simulink model "untitled"  (R2020a)
settings: Solver=VariableStepAuto  StartTime=0.0  StopTime=24  FixedStep=1e-6  MaxStep=1e-5  MinStep=1e-6  RelTol=1e-3
undefined symbols (not defined in the file): a, Acid, e_g, I_sc, k, Lead, N_p, N_s, q, R_s, R_sh, T_r, V_oc
libraries: powerlib x48, simulink x10, powerlib_meascontrol x6, electricdrivelib x1
settings Model: SimulationMode=accelerator  Creator=Tareeq  LastModifiedBy=Tareeq
settings SolverCC: AlgebraicLoopSolver=LineSearch

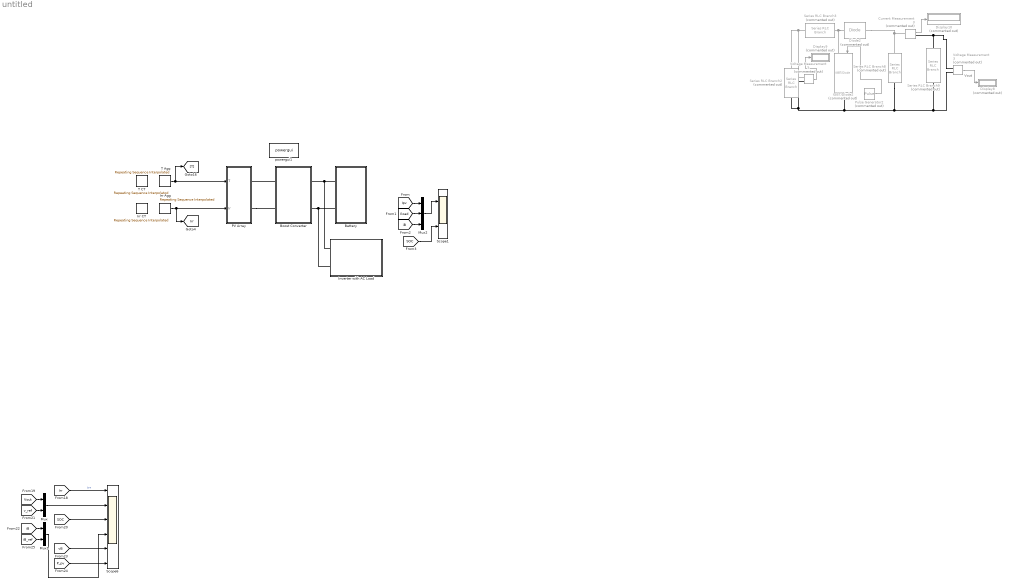
== system untitled ==
  note: Vout
  Battery : Subsystem
  Boost Converter : Subsystem
  Current Measurement3 : powerlib/Measurements/Current Measurement  Commented=on  PhasorSimulation=off  OutputType=Complex  PSBequivalent=0
  Diode2 : powerlib/Power Electronics/Diode  Commented=on  Ron=0.001  Lon=0  Vf=0.8  IC=0  UseSnubber=0  Rs=500  Cs=250e-9  Measurements=off
  Display10 : Display  Commented=on
  Display8 : Display  Commented=on
  Display9 : Display  Commented=on
  IGBT/Diode2 : powerlib/Power Electronics/IGBT//Diode  Commented=on  Ron=1e-3  Rs=inf  Cs=inf  Measurements=off
  Inverter with AC Load : Subsystem
  Irr Agg : simulink/Sources/Repeating Sequence Interpolated  OutValues="[0.412 0.412 0.395 0.395 0.407 0.407 0.332 0.332 0.375 0.375 0.384 0.384 0.345 0.345 0.994 0.994 462.1 462.1  804 804 922 922 973 973 996 996 1003 1003 1006 1006 988 988 881 881 828 828 338.9 338.9 240.5 240.5 0.015 0.015 0.119 0.119 0.375 0.375 0.291 0.291 ].'"  TimeValues=[0 1 1.01 2 2.01 3 3.01 4 4.01 5 5.01 6 6.01 7 7.01 8 8.01 9 9.01 10 10.01 11 11.01 12 12.01 13 13.01 14 14.01 15 15.01 16 16.01 17 17.01 18 18.01 19 19.01 20 20.01 21 21.01 22 22.02 23 23.01 24].'  LookUpMeth=Interpolation-Use End Values  tsamp=1e-5  OutMin=[]  OutMax=[]  OutDataTypeStr=double  OutputDataTypeScalingMode=double  OutDataType=fixdt(0,8)  OutScaling=2^-10
  Irr CT : simulink/Sources/Repeating Sequence Interpolated  OutValues=[0 0 0 0 0 0 0 0 0 0 2.6 2.6 53.2 53.2 151.6 151.6 270.1 270.1 383.6 383.6 450.5 450.5 480.4 480.4 474.3 474.3 443.6 443.6 375.2 375.2 288.4 288.4 200.3 200.3 122.3 122.3 61.3 61.3 14.1 14.1 0.1 0.1 0 0 0 0 0 0].'  TimeValues=[0 1 1.01 2 2.01 3 3.01 4 4.01 5 5.01 6 6.01 7 7.01 8 8.01 9 9.01 10 10.01 11 11.01 12 12.01 13 13.01 14 14.01 15 15.01 16 16.01 17 17.01 18 18.01 19 19.01 20 20.01 21 21.01 22 22.02 23 23.01 24].'  LookUpMeth=Interpolation-Use End Values  tsamp=1e-5  OutMin=[]  OutMax=[]  OutDataTypeStr=double  OutputDataTypeScalingMode=double  OutDataType=fixdt(0,8)  OutScaling=2^-10
  Mux : Mux  Inputs=2
  Mux1 : Mux  Inputs=2
  Mux2 : Mux  Inputs=3
  PV Array : Subsystem
  Pulse Generator2 : DiscretePulseGenerator  Commented=on  PulseType=Time based  Period=1/10000  PulseWidth=89
  Scope1 : Scope  NumInputPorts=2
  Scope6 : Scope  NumInputPorts=6
  Series RLC Branch2 : powerlib/Elements/Series RLC Branch  Commented=on  LConnTagsString=__new0  RConnTagsString=__new0  BranchType=C  Resistance=0.0001  Inductance=1e-3  SetiL0=off  InitialCurrent=0  Capacitance=2957.5e-6  Setx0=off  InitialVoltage=0  Measurements=None
  Series RLC Branch3 : powerlib/Elements/Series RLC Branch  Commented=on  LConnTagsString=__new0  RConnTagsString=__new0  BranchType=L  Resistance=0.0001  Inductance=153e-5  SetiL0=off  InitialCurrent=0  Capacitance=77.04e-6  Setx0=off  InitialVoltage=0  Measurements=None
  Series RLC Branch8 : powerlib/Elements/Series RLC Branch  Commented=on  LConnTagsString=__new0  RConnTagsString=__new0  BranchType=C  Resistance=0.0001  Inductance=780.60e-6  SetiL0=off  InitialCurrent=0  Capacitance=520.35e-6  Setx0=off  InitialVoltage=0  Measurements=None
  Series RLC Branch9 : powerlib/Elements/Series RLC Branch  Commented=on  LConnTagsString=__new0  RConnTagsString=__new0  BranchType=R  Resistance=173  Inductance=780.60e-6  SetiL0=off  InitialCurrent=0  Capacitance=2.09e-6  Setx0=off  InitialVoltage=0  Measurements=None
  T Agg : simulink/Sources/Repeating Sequence Interpolated  OutValues=[27.9 27.9 26.65 26.65 26.01 26.01 25.06 25.06 22.9 22.9 21.38 21.38 20.93 20.93 20.06 20.06 22.17 22.17 26.32 26.32 30.42 30.42 33.67 33.67 36.43 36.43 38.46 38.46 40.52 40.52 41.41 41.41 41.7 41.7 41.92 41.92 41.44 41.44 39.97 39.97 36.15 36.15 34.32 34.32 32.02 32.02 30.8 30.8].'  TimeValues=[0 1 1.01 2 2.01 3 3.01 4 4.01 5 5.01 6 6.01 7 7.01 8 8.01 9 9.01 10 10.01 11 11.01 12 12.01 13 13.01 14 14.01 15 15.01 16 16.01 17 17.01 18 18.01 19 19.01 20 20.01 21 21.01 22 22.01 23 23.01 24].'  LookUpMeth=Interpolation-Use End Values  tsamp=1e-5  OutMin=[]  OutMax=[]  OutDataTypeStr=double  OutputDataTypeScalingMode=double  OutDataType=fixdt(0,8)  OutScaling=2^-10
  T CT : simulink/Sources/Repeating Sequence Interpolated  OutValues=[16.07 16.07 15.8 15.8 15.52 15.52 15.29 15.29 15.07 15.07 14.88 14.88 14.88 14.88 15.39 15.39 16.53 16.53 18.11 18.11 19.4 19.4 20.28 20.28 20.79 20.79 21.08 21.08 21.21 21.21 21.10 21.10 20.72 20.72 19.98 19.98 18.88 18.88 17.94 17.94 17.35 17.35 16.99 16.99 16.65 16.65 16.35 16.35].'  TimeValues=[0 1 1.01 2 2.01 3 3.01 4 4.01 5 5.01 6 6.01 7 7.01 8 8.01 9 9.01 10 10.01 11 11.01 12 12.01 13 13.01 14 14.01 15 15.01 16 16.01 17 17.01 18 18.01 19 19.01 20 20.01 21 21.01 22 22.01 23 23.01 24].'  LookUpMeth=Interpolation-Use End Values  tsamp=1e-5  OutMin=[]  OutMax=[]  OutDataTypeStr=double  OutputDataTypeScalingMode=double  OutDataType=fixdt(0,8)  OutScaling=2^-10
  Voltage Measurement3 : powerlib/Measurements/Voltage Measurement  Commented=on  PhasorSimulation=off  OutputType=Complex  PSBequivalent=0
  Voltage Measurement5 : powerlib/Measurements/Voltage Measurement  Commented=on  PhasorSimulation=off  OutputType=Complex  PSBequivalent=0
  powergui1 : powerlib/powergui  Priority=1  SimulationMode=Continuous  SampleTime=1e-5  frequency=60  Iterations=50  frequencyindice=0  Pbase=100e6  ErrMax=1e-4  UnitsV=kV  UnitsW=MW  buscounter=0  FunctionMessages=off  echomessages=off  EnableUseOfTLC=off  CurrentSourceSwitches=off  DisableSnubberDevices=off  DisableRonSwitches=off  DisableVfSwitches=off  DisplayEquations=off  AutomaticDiscreteSolvers=off  SolverType=Tustin/Backward Euler (TBE)  Interpol=off  ExternalGateDelay=off  methode=off  Ts=100  x0status=blocks  SPID=on  SwTol=0  HookPort=off  NonlinearTolerance=1e-4  nMaxIteration=100  ContinueOnMaxIteration=off  RestoreLinks=warning  ResistiveCurrentMeasurement=off  Frange=[0:2:500]  Ylog=off  Xlog=on  ShowGrid=off  save=off  variable=ZData  structure=0  ZoomFFT=off  StartTime=0.0  cycles=1  DisplayStyle=1  fundamental=60  FreqAxis=off  MaxFrequency=1000  frequencyindicesteady=1  RmsSteady=1  display=off
  tag scope: Irr=global
  wires:
  [Irr] -> Scope6/1  "irr"
  [v_ref] -> Mux/2
  [iB] -> Mux1/1
  [iB_ref] -> Mux1/2
  [P_pv] -> Scope6/6
  Mux1/1 -> Scope6/4
  [SOC] -> Scope6/3
  Mux/1 -> Scope6/2
  [vB] -> Scope6/5
  [Vout] -> Mux/1
  Voltage Measurement5/1 -> Display9/1
  Voltage Measurement3/1 -> Display8/1
  Pulse Generator2/1 -> IGBT/Diode2/1
  Current Measurement3/1 -> Display10/1
  Irr Agg/1 -> [Irr], PV Array/2(Ir)
  T Agg/1 -> [T], PV Array/1(T)
  Mux2/1 -> Scope1/1
  [iB] -> Mux2/3
  [Iload] -> Mux2/2
  [Ipv] -> Mux2/1
  [SOC] -> Scope1/2
  connections:
  Current Measurement3/RConn1 -- Voltage Measurement3/LConn1 -- Series RLC Branch9/RConn1
  Series RLC Branch2/RConn1 -- Voltage Measurement5/LConn2 -- IGBT/Diode2/RConn1 -- Voltage Measurement3/LConn2 -- Series RLC Branch9/LConn1 -- Series RLC Branch8/RConn1
  Diode2/LConn1 -- Series RLC Branch3/LConn1 -- IGBT/Diode2/LConn1
  Diode2/RConn1 -- Series RLC Branch8/LConn1 -- Current Measurement3/LConn1
  Series RLC Branch3/RConn1 -- Voltage Measurement5/LConn1 -- Series RLC Branch2/LConn1
  Boost Converter/LConn1 -- PV Array/RConn1
  PV Array/RConn2 -- Boost Converter/LConn2
  Boost Converter/RConn2 -- Inverter with AC Load/LConn2 -- Battery/LConn2
  Boost Converter/RConn1 -- Inverter with AC Load/LConn1 -- Battery/LConn1

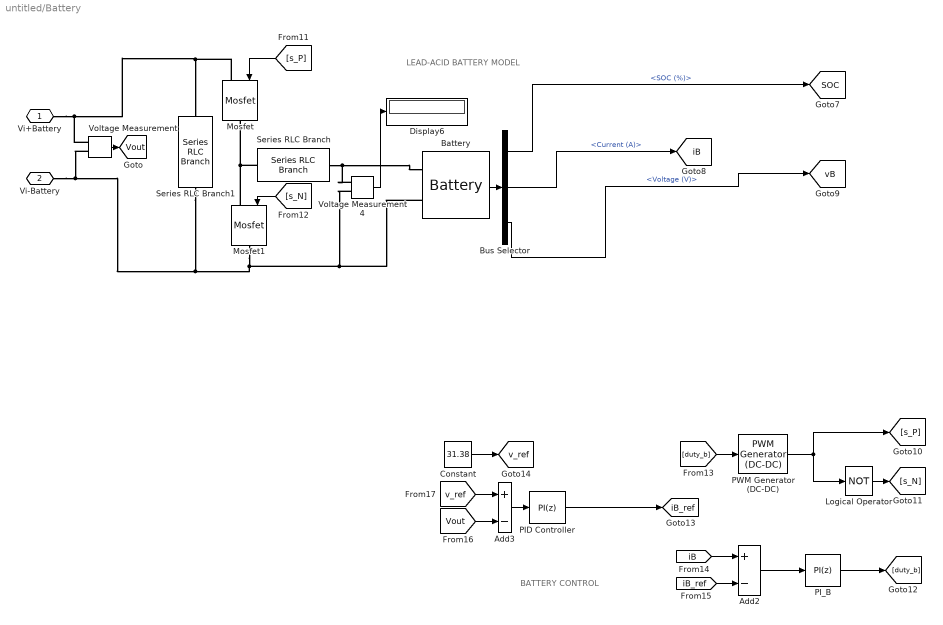
== system untitled/Battery ==
  note: LEAD-ACID BATTERY MODEL
  note: BATTERY CONTROL
  Add2 : Sum  Inputs=+-
  Add3 : Sum  Inputs=+-
  Battery : electricdrivelib/Extra Sources/Battery  BatType=Lead-Acid  ShowTempParam=off  ThermalPreset=no  ShowAgeParam=off  NomV=24  NomQ=400  SOC=100  Batt_Tr=1  PresetModel=on  MaxQ=416.6667  MinV=18  FullV=26.1316  Dis_rate=80  R=0.0006  Normal_OP=124.1111  expZone="[24.4342      1.33333]"  current=[6.5 13 32.5]  Units=Time  Tci=20  NomT=20  T2=-30  MaxQ2=4.8  FullV2=7.1  Normal_OP2=5.655  expZone2="[6.58           1]"  Rca=0.6  ti=2000  Dp=0  Neq0=0  Tsim=1e6  Ta1=25  Qeol=5.4*0.9  Reol=0.013333*1.2  Char_age=[2.3478, 3]  Dis_age=[2.3478, 10]  N1=1500  N2=10500  N3=1000  N4=1400  Ta2=45  N5=950
  Bus Selector : BusSelector  OutputSignals=SOC (%),Current (A),Voltage (V)
  Constant : Constant  Value=31.38
  Display6 : Display
  Logical Operator : Logic  Operator=NOT  Inputs=1  AllPortsSameDT=off  OutDataTypeStr=boolean
  Mosfet : powerlib/Power Electronics/Mosfet  Ron=0.1  Lon=0  Rd=0.01  Vfd=0  IC=0  Rs=1e5  Cs=inf  Measurements=off
  Mosfet1 : powerlib/Power Electronics/Mosfet  Ron=0.1  Lon=0  Rd=0.01  Vfd=0  IC=0  Rs=1e5  Cs=inf  Measurements=off
  PID Controller : simulink/Continuous/PID Controller  Controller=PI  Form=Parallel  TimeDomain=Discrete-time  UseExternalTs=off  SampleTime=50e-6  IntegratorMethod=Forward Euler  FilterMethod=Forward Euler  ControllerParametersSource=internal  P=0.05  I=100  D=0  UseFilter=on  N=100  TunerSelectOption=Transfer Function Based (PID Tuner App)  InitialConditionSource=internal  InitialConditionForIntegrator=1  InitialConditionForFilter=0  DifferentiatorICPrevScaledInput=0  ExternalReset=none  TrackingMode=off  Kt=1  LimitOutput=on  UpperSaturationLimit=80  LowerSaturationLimit=-80  LinearizeAsGain=on  AntiWindupMode=none  Kb=1  POutMin=[]  POutMax=[]  IOutMin=[]  IOutMax=[]  DOutMin=[]  DOutMax=[]  NOutMin=[]  NOutMax=[]  SumOutMin=[]  SumOutMax=[]  SaturationOutMin=[]  SaturationOutMax=[]  PParamMin=[]  PParamMax=[]  IParamMin=[]  IParamMax=[]  DParamMin=[]  DParamMax=[]  NParamMin=[]  NParamMax=[]  KbParamMin=[]  KbParamMax=[]  KtParamMin=[]  KtParamMax=[]  KbOutMin=[]  KbOutMax=[]  KtOutMin=[]  KtOutMax=[]  IntegratorOutMin=[]  IntegratorOutMax=[]  FilterOutMin=[]  FilterOutMax=[]  SumI1OutMin=[]  SumI1OutMax=[]  SumI2OutMin=[]  SumI2OutMax=[]  SumI3OutMin=[]  SumI3OutMax=[]  SumI4OutMin=[]  SumI4OutMax=[]  SumDOutMin=[]  SumDOutMax=[]  DifferentiatorOutMin=[]  DifferentiatorOutMax=[]  FilterDiffOutCoefMin=[]  FilterDiffOutCoefMax=[]  ReciprocalOutMin=[]  ReciprocalOutMax=[]  SumDenOutMin=[]  SumDenOutMax=[]  SumNumOutMin=[]  SumNumOutMax=[]  DivideOutMin=[]  DivideOutMax=[]  UdiffTsProdOutMin=[]  UdiffTsProdOutMax=[]  NTsProdOutMin=[]  NTsProdOutMax=[]  UintegralTsProdOutMin=[]  UintegralTsProdOutMax=[]  UngainTsProdOutMin=[]  UngainTsProdOutMax=[]  IntegratorContinuousStateAttributes=''  IntegratorStateMustResolveToSignalObject=off  IntegratorRTWStateStorageClass=Auto  FilterContinuousStateAttributes=''  FilterStateMustResolveToSignalObject=off  FilterRTWStateStorageClass=Auto  ParallelPVariant=InternalParameters  IdealPVariant=Disabled  IVariant=InternalParameters  DVariant=Disabled  IntegratorVariant=Discrete  SatVariant=Enabled  AWVariant=Passthrough  PCopyVariant=Disabled  TRVariant=Disabled  FdbkBlocksVariant=Forward  IdealPFdbkVariant=Disabled  SatFdbkVariant=Disabled  DerivativeFilterVariant=Disabled  NVariant=Disabled  NCopyVariant=Disabled_SignalSpec  FilterICVariant=Disabled  IntegratorICVariant=InternalICs  ExternalResetVariant=Disabled  TRSumVariant=Passthrough  SumFdbkVariant=Disabled  SumVariant=Sum_PI  TsampFilterVariant=InternalTs  TsampNgainVariant=Passthrough  TsampIntegralVariant=Passthrough
  PI_B : simulink/Continuous/PID Controller  Controller=PI  Form=Parallel  TimeDomain=Discrete-time  UseExternalTs=off  SampleTime=1e-5  IntegratorMethod=Forward Euler  FilterMethod=Forward Euler  ControllerParametersSource=internal  P=0.5  I=10  D=0  UseFilter=on  N=100  TunerSelectOption=Transfer Function Based (PID Tuner App)  InitialConditionSource=internal  InitialConditionForIntegrator=0  InitialConditionForFilter=0  DifferentiatorICPrevScaledInput=0  ExternalReset=none  TrackingMode=off  Kt=1  LimitOutput=on  UpperSaturationLimit=1  LowerSaturationLimit=0  LinearizeAsGain=off  AntiWindupMode=none  Kb=1  POutMin=[]  POutMax=[]  IOutMin=[]  IOutMax=[]  DOutMin=[]  DOutMax=[]  NOutMin=[]  NOutMax=[]  SumOutMin=[]  SumOutMax=[]  SaturationOutMin=[]  SaturationOutMax=[]  PParamMin=[]  PParamMax=[]  IParamMin=[]  IParamMax=[]  DParamMin=[]  DParamMax=[]  NParamMin=[]  NParamMax=[]  KbParamMin=[]  KbParamMax=[]  KtParamMin=[]  KtParamMax=[]  KbOutMin=[]  KbOutMax=[]  KtOutMin=[]  KtOutMax=[]  IntegratorOutMin=[]  IntegratorOutMax=[]  FilterOutMin=[]  FilterOutMax=[]  SumI1OutMin=[]  SumI1OutMax=[]  SumI2OutMin=[]  SumI2OutMax=[]  SumI3OutMin=[]  SumI3OutMax=[]  SumI4OutMin=[]  SumI4OutMax=[]  SumDOutMin=[]  SumDOutMax=[]  DifferentiatorOutMin=[]  DifferentiatorOutMax=[]  FilterDiffOutCoefMin=[]  FilterDiffOutCoefMax=[]  ReciprocalOutMin=[]  ReciprocalOutMax=[]  SumDenOutMin=[]  SumDenOutMax=[]  SumNumOutMin=[]  SumNumOutMax=[]  DivideOutMin=[]  DivideOutMax=[]  UdiffTsProdOutMin=[]  UdiffTsProdOutMax=[]  NTsProdOutMin=[]  NTsProdOutMax=[]  UintegralTsProdOutMin=[]  UintegralTsProdOutMax=[]  UngainTsProdOutMin=[]  UngainTsProdOutMax=[]  IntegratorContinuousStateAttributes=''  IntegratorStateMustResolveToSignalObject=off  IntegratorRTWStateStorageClass=Auto  FilterContinuousStateAttributes=''  FilterStateMustResolveToSignalObject=off  FilterRTWStateStorageClass=Auto  ParallelPVariant=InternalParameters  IdealPVariant=Disabled  IVariant=InternalParameters  DVariant=Disabled  IntegratorVariant=Discrete  SatVariant=Enabled  AWVariant=Passthrough  PCopyVariant=Disabled  TRVariant=Disabled  FdbkBlocksVariant=Forward  IdealPFdbkVariant=Disabled  SatFdbkVariant=Disabled  DerivativeFilterVariant=Disabled  NVariant=Disabled  NCopyVariant=Disabled_SignalSpec  FilterICVariant=Disabled  IntegratorICVariant=InternalICs  ExternalResetVariant=Disabled  TRSumVariant=Passthrough  SumFdbkVariant=Disabled  SumVariant=Sum_PI  TsampFilterVariant=InternalTs  TsampNgainVariant=Passthrough  TsampIntegralVariant=Passthrough
  PWM Generator (DC-DC) : powerlib_meascontrol/Pulse & Signal Generators/PWM Generator (DC-DC)  Fsw=10e3  Ts=1e-5
  Series RLC Branch : powerlib/Elements/Series RLC Branch  LConnTagsString=__new0  RConnTagsString=__new0  BranchType=RL  Resistance=0.005  Inductance=5.76e-4  SetiL0=off  InitialCurrent=0  Capacitance=0.5e-3  Setx0=off  InitialVoltage=0  Measurements=None
  Series RLC Branch1 : powerlib/Elements/Series RLC Branch  LConnTagsString=__new0  RConnTagsString=__new0  BranchType=RC  Resistance=1e-4  Inductance=780.60e-6  SetiL0=off  InitialCurrent=0  Capacitance=1e-6  Setx0=off  InitialVoltage=0  Measurements=None
  Voltage Measurement : powerlib/Measurements/Voltage Measurement  PhasorSimulation=off  OutputType=Complex  PSBequivalent=0
  Voltage Measurement4 : powerlib/Measurements/Voltage Measurement  PhasorSimulation=off  OutputType=Complex  PSBequivalent=0
  Vi+Battery : PMIOPort  Side=Left
  Vi-Battery : PMIOPort  Port=2  Side=Left
  tag scope: SOC=global, Vout=global, iB=global, iB_ref=global, vB=global, v_ref=global
  wires:
  Voltage Measurement4/1 -> Display6/1
  Bus Selector/3 -> [vB]  "<Voltage (V)>"
  [s_N] -> Mosfet1/1
  Bus Selector/2 -> [iB]  "<Current (A)>"
  [s_P] -> Mosfet/1
  Battery/1 -> Bus Selector/1
  [duty_b] -> PWM Generator (DC-DC)/1
  Constant/1 -> [v_ref]
  [iB] -> Add2/1
  [Vout] -> Add3/2
  [iB_ref] -> Add2/2
  Add3/1 -> PID Controller/1
  PI_B/1 -> [duty_b]
  [v_ref] -> Add3/1
  PWM Generator (DC-DC)/1 -> Logical Operator/1, [s_P]
  PID Controller/1 -> [iB_ref]
  Add2/1 -> PI_B/1
  Logical Operator/1 -> [s_N]
  Voltage Measurement/1 -> [Vout]
  Bus Selector/1 -> [SOC]  "<SOC (%)>"
  connections:
  Battery/LConn1 -- Series RLC Branch/RConn1 -- Voltage Measurement4/LConn1
  Mosfet/RConn1 -- Series RLC Branch/LConn1 -- Mosfet1/LConn1
  Mosfet/LConn1 -- Voltage Measurement/LConn1 -- Vi+Battery/RConn1 -- Series RLC Branch1/LConn1
  Battery/LConn2 -- Voltage Measurement/LConn2 -- Vi-Battery/RConn1 -- Series RLC Branch1/RConn1 -- Mosfet1/RConn1 -- Voltage Measurement4/LConn2

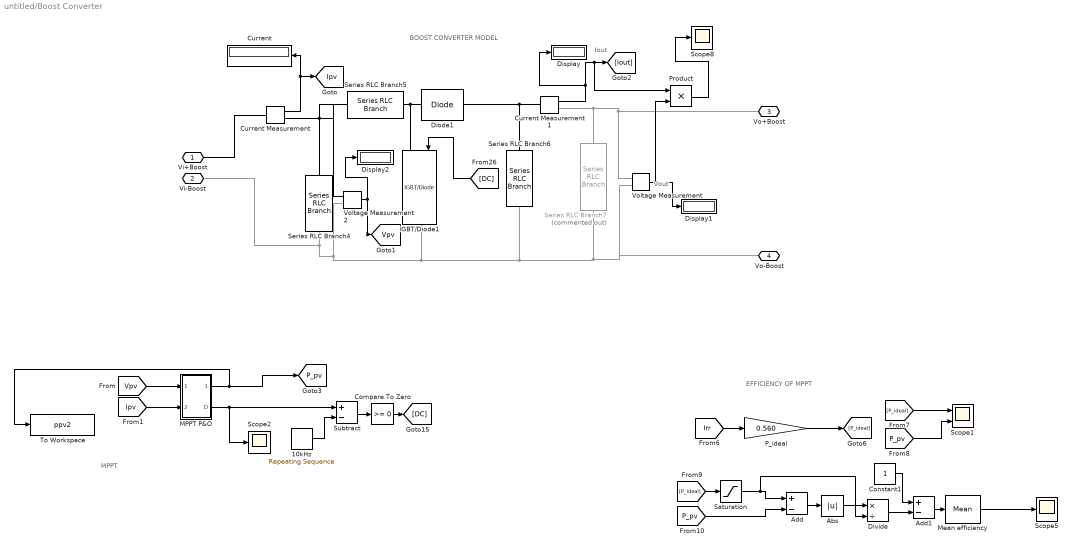
== system untitled/Boost Converter ==
  note: Iout
  note: Vout
  note: BOOST CONVERTER MODEL
  note: MPPT
  note: EFFICIENCY OF MPPT
  10kHz : simulink/Sources/Repeating Sequence  rep_seq_t=[0 1e-4]  rep_seq_y=[0 1]
  Abs : Abs
  Add : Sum  Inputs=+-
  Add1 : Sum  Inputs=+-
  Compare To Zero : simulink/Logic and Bit Operations/Compare To Zero  relop=>=  OutDataTypeStr=boolean
  Constant1 : Constant
  Current : Display
  Current Measurement : powerlib/Measurements/Current Measurement  PhasorSimulation=off  OutputType=Complex  PSBequivalent=0
  Current Measurement1 : powerlib/Measurements/Current Measurement  PhasorSimulation=off  OutputType=Complex  PSBequivalent=0
  Diode1 : powerlib/Power Electronics/Diode  Ron=0.001  Lon=0  Vf=0.8  IC=0  UseSnubber=0  Rs=500  Cs=250e-9  Measurements=off
  Display : Display
  Display1 : Display
  Display2 : Display
  Divide : Product  Inputs=*/
  IGBT/Diode1 : powerlib/Power Electronics/IGBT//Diode  Ron=1e-3  Rs=1e5  Cs=inf  Measurements=off
  MPPT P&O : Subsystem
  Mean efficiency : powerlib_meascontrol/Measurements/Mean  Freq=50  Vinit=0  Ts=500e-6
  P_ideal : Gain  Gain=0.560
  Product : Product
  Saturation : Saturate  UpperLimit=1000  LowerLimit=0
  Scope1 : Scope  NumInputPorts=2
  Scope2 : Scope
  Scope5 : Scope
  Scope8 : Scope
  Series RLC Branch4 : powerlib/Elements/Series RLC Branch  LConnTagsString=__new0  RConnTagsString=__new0  BranchType=C  Resistance=0.0001  Inductance=1e-3  SetiL0=off  InitialCurrent=0  Capacitance=308.19e-6  Setx0=off  InitialVoltage=0  Measurements=None
  Series RLC Branch5 : powerlib/Elements/Series RLC Branch  LConnTagsString=__new0  RConnTagsString=__new0  BranchType=L  Resistance=0.0001  Inductance=195.51e-6  SetiL0=off  InitialCurrent=0  Capacitance=77.04e-6  Setx0=off  InitialVoltage=0  Measurements=None
  Series RLC Branch6 : powerlib/Elements/Series RLC Branch  LConnTagsString=__new0  RConnTagsString=__new0  BranchType=C  Resistance=0.0001  Inductance=780.60e-6  SetiL0=off  InitialCurrent=0  Capacitance=834.39e-5  Setx0=off  InitialVoltage=0  Measurements=None
  Series RLC Branch7 : powerlib/Elements/Series RLC Branch  Commented=on  LConnTagsString=__new0  RConnTagsString=__new0  BranchType=R  Resistance=3.9545  Inductance=780.60e-6  SetiL0=off  InitialCurrent=0  Capacitance=2.09e-6  Setx0=off  InitialVoltage=0  Measurements=None
  Subtract : Sum  Inputs=+-
  To Workspace : ToWorkspace  VariableName=ppv2  SaveFormat=Timeseries  SampleTime=-1
  Voltage Measurement : powerlib/Measurements/Voltage Measurement  PhasorSimulation=off  OutputType=Complex  PSBequivalent=0
  Voltage Measurement2 : powerlib/Measurements/Voltage Measurement  PhasorSimulation=off  OutputType=Complex  PSBequivalent=0
  Vi+Boost : PMIOPort  Side=Left
  Vi-Boost : PMIOPort  Port=2  Side=Left
  Vo+Boost : PMIOPort  Port=3  Side=Right
  Vo-Boost : PMIOPort  Port=4  Side=Right
  tag scope: Ipv=global, P_pv=global, Vpv=global
  wires:
  Product/1 -> Scope8/1
  Voltage Measurement/1 -> Product/2, Display1/1
  Current Measurement/1 -> Current/1, [Ipv]
  Current Measurement1/1 -> Product/1, [Iout], Display/1
  Voltage Measurement2/1 -> [Vpv], Display2/1
  [DC] -> IGBT/Diode1/1
  MPPT P&O/2(D) -> Scope2/1, Subtract/1
  Compare To Zero/1 -> [DC]
  Subtract/1 -> Compare To Zero/1
  MPPT P&O/1(Ppv) -> [P_pv], To Workspace/1
  10kHz/1 -> Subtract/2
  [Ipv] -> MPPT P&O/2(Ipv)
  [Vpv] -> MPPT P&O/1(Vpv)
  P_ideal/1 -> [P_ideal]
  [P_ideal] -> Scope1/1
  Add/1 -> Abs/1
  [Irr] -> P_ideal/1
  Saturation/1 -> Divide/2, Add/1
  Mean efficiency/1 -> Scope5/1
  Add1/1 -> Mean efficiency/1
  Abs/1 -> Divide/1
  [P_pv] -> Add/2
  Divide/1 -> Add1/2
  [P_pv] -> Scope1/2
  [P_ideal] -> Saturation/1
  Constant1/1 -> Add1/1
  connections:
  Current Measurement/RConn1 -- Series RLC Branch5/RConn1 -- Voltage Measurement2/LConn1 -- Series RLC Branch4/LConn1
  Series RLC Branch6/LConn1 -- Current Measurement1/LConn1 -- Diode1/RConn1
  Series RLC Branch7/RConn1 -- Vo+Boost/RConn1 -- Voltage Measurement/LConn1 -- Current Measurement1/RConn1
  Series RLC Branch7/LConn1 -- Vo-Boost/RConn1 -- Voltage Measurement/LConn2 -- Series RLC Branch6/RConn1 -- IGBT/Diode1/RConn1 -- Voltage Measurement2/LConn2 -- Vi-Boost/RConn1 -- Series RLC Branch4/RConn1
  Diode1/LConn1 -- Series RLC Branch5/LConn1 -- IGBT/Diode1/LConn1
  Current Measurement/LConn1 -- Vi+Boost/RConn1

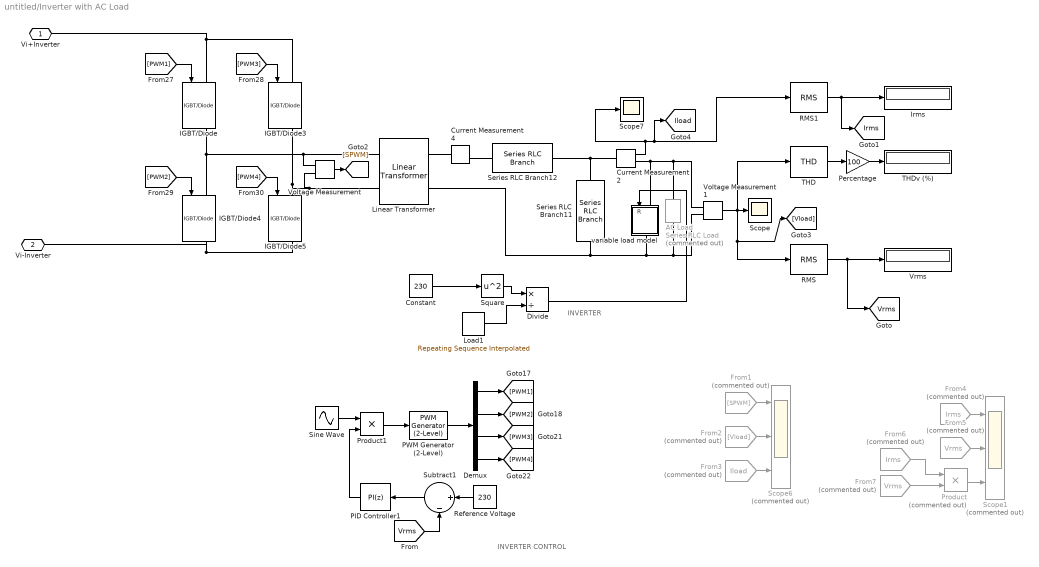
== system untitled/Inverter with AC Load ==
  note: INVERTER
  note: INVERTER CONTROL
  " variable load model" : Subsystem
  AC Load : powerlib/Elements/Series RLC Load  Commented=on  LConnTagsString=a  RConnTagsString=__new0  NominalVoltage=230  NominalFrequency=50  ActivePower=370  InductivePower=0  CapacitivePower=0  Setx0=off  InitialVoltage=0  SetiL0=off  InitialCurrent=0  Measurements=Branch voltage and current  LoadType=constant Z
  Constant : Constant  Value=230
  Current Measurement2 : powerlib/Measurements/Current Measurement  PhasorSimulation=off  OutputType=Complex  PSBequivalent=0
  Current Measurement4 : powerlib/Measurements/Current Measurement  PhasorSimulation=off  OutputType=Complex  PSBequivalent=0
  Demux : Demux
  Divide : Product  Inputs=*/
  From1 : From  Commented=on  GotoTag=SPWM
  From2 : From  Commented=on  GotoTag=Vload
  From3 : From  Commented=on  GotoTag=Iload
  From4 : From  Commented=on  GotoTag=Irms  TagVisibility=global
  From5 : From  Commented=on  GotoTag=Vrms  TagVisibility=global
  From6 : From  Commented=on  GotoTag=Irms  TagVisibility=global
  From7 : From  Commented=on  GotoTag=Vrms  TagVisibility=global
  IGBT/Diode{,3..5} (4 alike) : powerlib/Power Electronics/IGBT//Diode  Ron=1e-3  Rs=1e5  Cs=inf  Measurements=on
  Irms : Display
  Linear Transformer : powerlib/Elements/Linear Transformer  UNITS=SI  NominalPower=[ 800 50 ]  winding1=[12 0 0]  winding2=[230 0 0]  ThreeWindings=off  winding3=[3.15e+05 2.4806e+05 31584]  RmLm=[500 500]  Measurements=None  DataType=on
  Load1 : simulink/Sources/Repeating Sequence Interpolated  OutValues=[0.01 0.01 0.01 0.01 0.01 0.01 0.01 0.01 0.01 0.01 0.01 0.01 187.5 187.5 275 275 298.125 298.125 298.125 298.125 371.875 371.875 371.875 371.875 318.75 318.75 193.75 193.75 66.875 66.875 66.875 66.875 0.01 0.01 0.01 0.01 0.01 0.01 0.01 0.01 0.01 0.01 43.75 43.75 43.75 43.75 0 0].'  TimeValues=[0 1 1.01 2 2.01 3 3.01 4 4.01 5 5.01 6 6.01 7 7.01 8 8.01 9 9.01 10 10.01 11 11.01 12 12.01 13 13.01 14 14.01 15 15.01 16 16.01 17 17.01 18 18.01 19 19.01 20 20.01 21 21.01 22 22.01 23 23.01 24].'  LookUpMeth=Interpolation-Use End Values  tsamp=1e-5  OutMin=[]  OutMax=[]  OutDataTypeStr=double  OutputDataTypeScalingMode=double  OutDataType=fixdt(0,8)  OutScaling=2^-10
  PID Controller1 : simulink/Continuous/PID Controller  Controller=PI  Form=Parallel  TimeDomain=Discrete-time  UseExternalTs=off  SampleTime=200e-6  IntegratorMethod=Forward Euler  FilterMethod=Forward Euler  ControllerParametersSource=internal  P=6.9e-4  I=0.091  D=0  UseFilter=on  N=100  TunerSelectOption=Transfer Function Based (PID Tuner App)  InitialConditionSource=internal  InitialConditionForIntegrator=0  InitialConditionForFilter=0  DifferentiatorICPrevScaledInput=0  ExternalReset=none  TrackingMode=off  Kt=1  LimitOutput=off  UpperSaturationLimit=inf  LowerSaturationLimit=-inf  LinearizeAsGain=on  AntiWindupMode=none  Kb=1  POutMin=[]  POutMax=[]  IOutMin=[]  IOutMax=[]  DOutMin=[]  DOutMax=[]  NOutMin=[]  NOutMax=[]  SumOutMin=[]  SumOutMax=[]  SaturationOutMin=[]  SaturationOutMax=[]  PParamMin=[]  PParamMax=[]  IParamMin=[]  IParamMax=[]  DParamMin=[]  DParamMax=[]  NParamMin=[]  NParamMax=[]  KbParamMin=[]  KbParamMax=[]  KtParamMin=[]  KtParamMax=[]  KbOutMin=[]  KbOutMax=[]  KtOutMin=[]  KtOutMax=[]  IntegratorOutMin=[]  IntegratorOutMax=[]  FilterOutMin=[]  FilterOutMax=[]  SumI1OutMin=[]  SumI1OutMax=[]  SumI2OutMin=[]  SumI2OutMax=[]  SumI3OutMin=[]  SumI3OutMax=[]  SumI4OutMin=[]  SumI4OutMax=[]  SumDOutMin=[]  SumDOutMax=[]  DifferentiatorOutMin=[]  DifferentiatorOutMax=[]  FilterDiffOutCoefMin=[]  FilterDiffOutCoefMax=[]  ReciprocalOutMin=[]  ReciprocalOutMax=[]  SumDenOutMin=[]  SumDenOutMax=[]  SumNumOutMin=[]  SumNumOutMax=[]  DivideOutMin=[]  DivideOutMax=[]  UdiffTsProdOutMin=[]  UdiffTsProdOutMax=[]  NTsProdOutMin=[]  NTsProdOutMax=[]  UintegralTsProdOutMin=[]  UintegralTsProdOutMax=[]  UngainTsProdOutMin=[]  UngainTsProdOutMax=[]  IntegratorContinuousStateAttributes=''  IntegratorStateMustResolveToSignalObject=off  IntegratorRTWStateStorageClass=Auto  FilterContinuousStateAttributes=''  FilterStateMustResolveToSignalObject=off  FilterRTWStateStorageClass=Auto  ParallelPVariant=InternalParameters  IdealPVariant=Disabled  IVariant=InternalParameters  DVariant=Disabled  IntegratorVariant=Discrete  SatVariant=Disabled  AWVariant=Passthrough  PCopyVariant=Disabled  TRVariant=Disabled  FdbkBlocksVariant=Forward  IdealPFdbkVariant=Disabled  SatFdbkVariant=Disabled  DerivativeFilterVariant=Disabled  NVariant=Disabled  NCopyVariant=Disabled_SignalSpec  FilterICVariant=Disabled  IntegratorICVariant=InternalICs  ExternalResetVariant=Disabled  TRSumVariant=Passthrough  SumFdbkVariant=Disabled  SumVariant=Sum_PI  TsampFilterVariant=InternalTs  TsampNgainVariant=Passthrough  TsampIntegralVariant=Passthrough
  PWM Generator (2-Level) : powerlib_meascontrol/Pulse & Signal Generators/PWM Generator (2-Level)  ModulatorType=Single-phase full-bridge (4 pulses)  ModulatorMode=Unsynchronized  Fc=200*50  Pc=90  nF=27  MinMax="[ -1  1 ]"  SamplingTechnique=Natural  ModulatingSignals=off  m=0.718  Freq=50  Phase=0  Ts=0  ShowCarrierOutport=off
  Percentage : Gain  Gain=100
  Product : Product  Commented=on
  Product1 : Product
  RMS : powerlib_meascontrol/Measurements/RMS  TrueRMS=on  Freq=50  RMSInit=0  Ts=0
  RMS1 : powerlib_meascontrol/Measurements/RMS  TrueRMS=on  Freq=50  RMSInit=0  Ts=0
  Reference Voltage : Constant  Value=230
  Scope : Scope
  Scope1 : Scope  Commented=on  NumInputPorts=3
  Scope6 : Scope  Commented=on  NumInputPorts=3
  Scope7 : Scope
  Series RLC Branch11 : powerlib/Elements/Series RLC Branch  LConnTagsString=__new0  RConnTagsString=__new0  BranchType=RC  Resistance=0.0042  Inductance=1e-3  SetiL0=off  InitialCurrent=0  Capacitance=31.76e-7  Setx0=off  InitialVoltage=0  Measurements=None
  Series RLC Branch12 : powerlib/Elements/Series RLC Branch  LConnTagsString=__new0  RConnTagsString=__new0  BranchType=RL  Resistance=0.001  Inductance=797.53e-5  SetiL0=off  InitialCurrent=0  Capacitance=1e-6  Setx0=off  InitialVoltage=0  Measurements=None
  Sine Wave : Sin  Frequency=314  SampleTime=0
  Square : Math  Operator=square  SaturateOnIntegerOverflow=on
  Subtract1 : Sum  Inputs=|||+||-
  THD : powerlib_meascontrol/Measurements/THD  Freq=50  Ts=0
  THDv (%) : Display
  Voltage Measurement : powerlib/Measurements/Voltage Measurement  PhasorSimulation=off  OutputType=Complex  PSBequivalent=0
  Voltage Measurement1 : powerlib/Measurements/Voltage Measurement  PhasorSimulation=off  OutputType=Complex  PSBequivalent=0
  Vrms : Display
  Vi+Inverter : PMIOPort  Side=Left
  Vi-Inverter : PMIOPort  Port=2  Side=Left
  tag scope: Iload=global, Irms=global, Vrms=global
  wires:
  THD/1 -> Percentage/1
  [PWM3] -> IGBT/Diode3/1
  Demux/3 -> [PWM3]
  [PWM4] -> IGBT/Diode5/1
  Current Measurement2/1 -> [Iload], RMS1/1, Scope7/1
  [PWM1] -> IGBT/Diode/1
  PID Controller1/1 -> Product1/2
  Demux/1 -> [PWM1]
  Voltage Measurement1/1 -> [Vload], RMS/1, THD/1, Scope/1
  Percentage/1 -> THDv (%)/1
  Demux/4 -> [PWM4]
  Sine Wave/1 -> Product1/1
  [Vrms] -> Subtract1/2
  RMS/1 -> [Vrms], Vrms/1
  Reference Voltage/1 -> Subtract1/1
  PWM Generator (2-Level)/1 -> Demux/1
  Product1/1 -> PWM Generator (2-Level)/1
  Subtract1/1 -> PID Controller1/1
  RMS1/1 -> Irms/1, [Irms]
  [PWM2] -> IGBT/Diode4/1
  Demux/2 -> [PWM2]
  Voltage Measurement/1 -> [SPWM]
  From3/1 -> Scope6/3
  From2/1 -> Scope6/2
  From1/1 -> Scope6/1
  From5/1 -> Scope1/2
  From4/1 -> Scope1/1
  Product/1 -> Scope1/3
  From6/1 -> Product/1
  From7/1 -> Product/2
  Square/1 -> Divide/1
  Divide/1 -> " variable load model"/1(R)
  Load1/1 -> Divide/2
  Constant/1 -> Square/1
  connections:
  Linear Transformer/RConn2 -- Voltage Measurement1/LConn2 -- AC Load/RConn1 -- " variable load model"/RConn1 -- Series RLC Branch11/RConn1
  IGBT/Diode5/RConn1 -- Vi-Inverter/RConn1 -- IGBT/Diode4/RConn1
  IGBT/Diode3/LConn1 -- Vi+Inverter/RConn1 -- IGBT/Diode/LConn1
  Voltage Measurement1/LConn1 -- AC Load/LConn1 -- " variable load model"/LConn1 -- Current Measurement2/RConn1
  Current Measurement4/LConn1 -- Linear Transformer/RConn1
  Series RLC Branch11/LConn1 -- Current Measurement2/LConn1 -- Series RLC Branch12/RConn1
  IGBT/Diode/RConn1 -- Linear Transformer/LConn1 -- Voltage Measurement/LConn1 -- IGBT/Diode4/LConn1
  Series RLC Branch12/LConn1 -- Current Measurement4/RConn1
  IGBT/Diode5/LConn1 -- Voltage Measurement/LConn2 -- Linear Transformer/LConn2 -- IGBT/Diode3/RConn1

== system untitled/PV Array ==
  T : Inport
  Ir : Inport  Port=2
  Current Measurement : powerlib/Measurements/Current Measurement  PhasorSimulation=off  OutputType=Complex  PSBequivalent=0
  Display : Display
  Display1 : Display
  PV Module 1 : Subsystem
  PV Module 2 : Subsystem
  Voltage Measurement : powerlib/Measurements/Voltage Measurement  PhasorSimulation=off  OutputType=Complex  PSBequivalent=0
  Vo+PV : PMIOPort  Side=Right
  Vo-PV : PMIOPort  Port=2  Side=Right
  wires:
  T/1 -> PV Module 2/1(T), PV Module 1/1(T)
  Ir/1 -> PV Module 2/2(Ir), PV Module 1/2(Ir)
  Current Measurement/1 -> Display/1
  Voltage Measurement/1 -> Display1/1
  connections:
  PV Module 1/RConn1 -- Current Measurement/LConn1 -- PV Module 2/RConn1
  PV Module 2/RConn2 -- Voltage Measurement/LConn2 -- Vo-PV/RConn1 -- PV Module 1/RConn2
  Vo+PV/RConn1 -- Voltage Measurement/LConn1 -- Current Measurement/RConn1

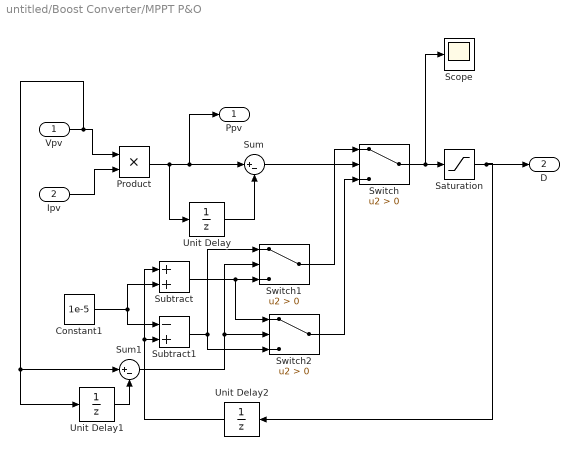
== system untitled/Boost Converter/MPPT P&O ==
  Vpv : Inport
  Ipv : Inport  Port=2
  Constant1 : Constant  Value=1e-5
  Product : Product
  Saturation : Saturate  UpperLimit=1  LowerLimit=0
  Scope : Scope
  Subtract : Sum
  Subtract1 : Sum  Inputs=-+
  Sum : Sum  Inputs=|+-
  Sum1 : Sum  Inputs=|+-
  Switch : Switch  Criteria=u2 > Threshold
  Switch1 : Switch  Criteria=u2 > Threshold
  Switch2 : Switch  Criteria=u2 > Threshold
  Unit Delay : UnitDelay  SampleTime=-1  HasFrameUpgradeWarning=on
  Unit Delay1 : UnitDelay  SampleTime=-1  HasFrameUpgradeWarning=on
  Unit Delay2 : UnitDelay  SampleTime=-1  HasFrameUpgradeWarning=on
  Ppv : Outport
  D : Outport  Port=2
  wires:
  Product/1 -> Ppv/1, Sum/1, Unit Delay/1
  Constant1/1 -> Subtract1/1, Subtract/2
  Saturation/1 -> D/1, Unit Delay2/1
  Vpv/1 -> Product/1, Sum1/1, Unit Delay1/1
  Sum1/1 -> Switch2/2, Switch1/2
  Switch1/1 -> Switch/1
  Sum/1 -> Switch/2
  Unit Delay1/1 -> Sum1/2
  Subtract1/1 -> Switch2/3, Switch1/1
  Unit Delay2/1 -> Subtract/1, Subtract1/2
  Subtract/1 -> Switch2/1, Switch1/3
  Ipv/1 -> Product/2
  Unit Delay/1 -> Sum/2
  Switch2/1 -> Switch/3
  Switch/1 -> Scope/1, Saturation/1

== system untitled/Inverter with AC Load/ variable load model ==
  R : Inport
  Abs : Abs  SampleTime=1e-03
  Controlled Current Source : powerlib/Electrical Sources/Controlled Current Source  Initialize=on  Source_Type=AC  Amplitude=0  Phase=0  Frequency=0  Measurements=None
  Product : Product
  Product2 : Product  Inputs=/*  RndMeth=Zero
  Sign : Signum
  Vab_load1 : powerlib/Measurements/Voltage Measurement  Tag=PoWeRsYsTeMmEaSuReMeNt  PhasorSimulation=off  OutputType=Magnitude  PSBequivalent=0
  short circuit : Saturate  UpperLimit=1000  LowerLimit=0.0001
  - : PMIOPort  Side=Right
  + : PMIOPort  Port=2  Side=Left
  wires:
  Product/1 -> Controlled Current Source/1
  short circuit/1 -> Product2/1
  Product2/1 -> Product/1
  R/1 -> Sign/1, Abs/1
  Sign/1 -> Product/2
  Abs/1 -> short circuit/1
  Vab_load1/1 -> Product2/2
  connections:
  Controlled Current Source/LConn1 -- Vab_load1/LConn1 -- -/RConn1
  Controlled Current Source/RConn1 -- +/RConn1 -- Vab_load1/LConn2

== system untitled/PV Array/PV Module 1 ==
  T : Inport
  Ir : Inport  Port=2
  CCS : powerlib/Electrical Sources/Controlled Current Source  Initialize=on  Source_Type=AC  Amplitude=0  Phase=0  Frequency=0  Measurements=None
  Diode : powerlib/Power Electronics/Diode  Ron=0.001  Lon=0  Vf=0.8  IC=0  UseSnubber=0  Rs=500  Cs=250e-9  Measurements=off
  PV Module : Subsystem  InitFcn=|
      | I_sc=9.45;
      | V_oc=39.12;
      | V_mp=31.38;
      | I_mp=8.93;
      | N_s=60;
      | N_p=1;
      | T_r=298.15;
      | q = 1.6e-19;
      | k = 1.3815e-23;
      | R_sh= 1000;
      | R_s = 0.001;
      | dV_dI_oc = -0.487;
      | a =1.725;
      | e_g = 1.1;
  Vo : powerlib/Measurements/Voltage Measurement  PhasorSimulation=off  OutputType=Complex  PSBequivalent=0
  + : PMIOPort  Tag=PMCPort  Side=Right
  - : PMIOPort  Tag=PMCPort  Port=2  Side=Right
  wires:
  Vo/1 -> PV Module/3(Vm)
  PV Module/1(I) -> CCS/1
  Ir/1 -> PV Module/2(Ir)
  T/1 -> PV Module/1(T)
  connections:
  Vo/LConn1 -- Diode/RConn1 -- CCS/RConn1 -- +/RConn1
  Vo/LConn2 -- Diode/LConn1 -- CCS/LConn1 -- -/RConn1

== system untitled/PV Array/PV Module 2 ==
  T : Inport
  Ir : Inport  Port=2
  CCS : powerlib/Electrical Sources/Controlled Current Source  Initialize=on  Source_Type=AC  Amplitude=0  Phase=0  Frequency=0  Measurements=None
  Diode : powerlib/Power Electronics/Diode  Ron=0.001  Lon=0  Vf=0.8  IC=0  UseSnubber=0  Rs=500  Cs=250e-9  Measurements=off
  PV Module : Subsystem  InitFcn=|
      | I_sc=9.45;
      | V_oc=39.12;
      | V_mp=31.38;
      | I_mp=8.93;
      | N_s=60;
      | N_p=1;
      | T_r=298.15;
      | q = 1.6e-19;
      | k = 1.3815e-23;
      | R_sh= 1000;
      | R_s = 0.001;
      | dV_dI_oc = -0.487;
      | a =1.725;
      | e_g = 1.1;
  Vo : powerlib/Measurements/Voltage Measurement  PhasorSimulation=off  OutputType=Complex  PSBequivalent=0
  + : PMIOPort  Tag=PMCPort  Side=Right
  - : PMIOPort  Tag=PMCPort  Port=2  Side=Right
  wires:
  Vo/1 -> PV Module/3(Vm)
  PV Module/1(I) -> CCS/1
  Ir/1 -> PV Module/2(Ir)
  T/1 -> PV Module/1(T)
  connections:
  Vo/LConn1 -- +/RConn1 -- CCS/RConn1 -- Diode/RConn1
  CCS/LConn1 -- -/RConn1 -- Vo/LConn2 -- Diode/LConn1

== system untitled/PV Array/PV Module 1/PV Module ==
  T : Inport
  Ir : Inport  Port=2
  Vm : Inport  Port=3
  Add : Sum
  Constant : Constant  Value=273.15
  Current through shunt resistor : Subsystem
  Output current : Subsystem
  Photon current : Subsystem
  Reverse saturation current : Subsystem
  Saturation current : Subsystem
  I : Outport
  wires:
  Reverse saturation current/1(Vt) -> Output current/2(Vt)
  Saturation current/1(Io) -> Output current/3(Io)
  Photon current/1(Iph) -> Output current/4(Iph)
  Ir/1 -> Photon current/2(Ir)
  Output current/1(I) -> I/1, Current through shunt resistor/2(I)
  Add/1 -> Photon current/1(T), Reverse saturation current/1(T), Saturation current/1(T)
  Vm/1 -> Current through shunt resistor/1(V), Output current/1(V)
  Current through shunt resistor/1(Ish) -> Output current/5(Ish)
  Constant/1 -> Add/2
  T/1 -> Add/1
  Reverse saturation current/2(Irs) -> Saturation current/2(Irs)

== system untitled/PV Array/PV Module 2/PV Module ==
  T : Inport
  Ir : Inport  Port=2
  Vm : Inport  Port=3
  Add : Sum
  Constant : Constant  Value=273.15
  Current through shunt resistor : Subsystem
  Output current : Subsystem
  Photon current : Subsystem
  Reverse saturation current : Subsystem
  Saturation current : Subsystem
  I : Outport
  wires:
  Reverse saturation current/1(Vt) -> Output current/2(Vt)
  Saturation current/1(Io) -> Output current/3(Io)
  Photon current/1(Iph) -> Output current/4(Iph)
  Ir/1 -> Photon current/2(Ir)
  Output current/1(I) -> I/1, Current through shunt resistor/2(I)
  Add/1 -> Photon current/1(T), Reverse saturation current/1(T), Saturation current/1(T)
  Vm/1 -> Current through shunt resistor/1(V), Output current/1(V)
  Current through shunt resistor/1(Ish) -> Output current/5(Ish)
  Constant/1 -> Add/2
  T/1 -> Add/1
  Reverse saturation current/2(Irs) -> Saturation current/2(Irs)

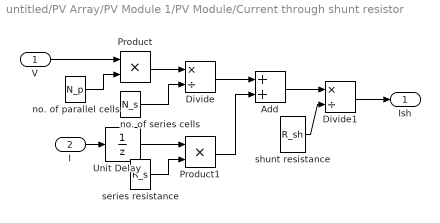
== system untitled/PV Array/PV Module 1/PV Module/Current through shunt resistor ==
  V : Inport
  I : Inport  Port=2
  Add : Sum
  Divide : Product  Inputs=*/
  Divide1 : Product  Inputs=*/
  Product : Product
  Product1 : Product
  Unit Delay : UnitDelay  SampleTime=-1  HasFrameUpgradeWarning=on
  no. of parallel cells : Constant  Value=N_p
  no. of series cells : Constant  Value=N_s
  series resistance : Constant  Value=R_s
  shunt resistance : Constant  Value=R_sh
  Ish : Outport
  wires:
  no. of parallel cells/1 -> Product/2
  V/1 -> Product/1
  Divide1/1 -> Ish/1
  Divide/1 -> Add/1
  Product1/1 -> Add/2
  series resistance/1 -> Product1/2
  shunt resistance/1 -> Divide1/2
  no. of series cells/1 -> Divide/2
  Add/1 -> Divide1/1
  Product/1 -> Divide/1
  I/1 -> Unit Delay/1
  Unit Delay/1 -> Product1/1

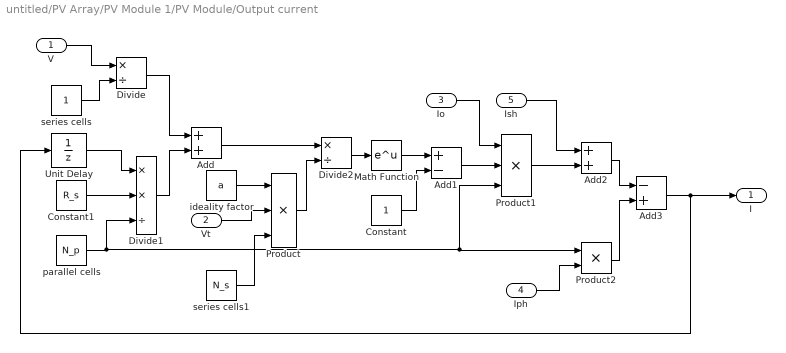
== system untitled/PV Array/PV Module 1/PV Module/Output current ==
  V : Inport
  Vt : Inport  Port=2
  Io : Inport  Port=3
  Iph : Inport  Port=4
  Ish : Inport  Port=5
  Add : Sum
  Add1 : Sum  Inputs=+-
  Add2 : Sum
  Add3 : Sum  Inputs=-+
  Constant : Constant
  Constant1 : Constant  Value=R_s
  Divide : Product  Inputs=*/
  Divide1 : Product  Inputs=**/
  Divide2 : Product  Inputs=*/
  Math Function : Math  SaturateOnIntegerOverflow=on
  Product : Product  Inputs=3
  Product1 : Product  Inputs=3
  Product2 : Product
  Unit Delay : UnitDelay  SampleTime=-1  HasFrameUpgradeWarning=on
  ideality factor : Constant  Value=a
  parallel cells : Constant  Value=N_p
  series cells : Constant
  series cells1 : Constant  Value=N_s
  I : Outport
  wires:
  V/1 -> Divide/1
  Constant/1 -> Add1/2
  parallel cells/1 -> Product2/1, Product1/3, Divide1/3
  Vt/1 -> Product/2
  Add2/1 -> Add3/1
  Ish/1 -> Add2/1
  Product/1 -> Divide2/2
  Divide1/1 -> Add/2
  Divide2/1 -> Math Function/1
  Iph/1 -> Product2/2
  Math Function/1 -> Add1/1
  ideality factor/1 -> Product/1
  Constant1/1 -> Divide1/2
  Add/1 -> Divide2/1
  Product2/1 -> Add3/2
  series cells/1 -> Divide/2
  Divide/1 -> Add/1
  Add1/1 -> Product1/2
  Product1/1 -> Add2/2
  Io/1 -> Product1/1
  Add3/1 -> Unit Delay/1, I/1
  Unit Delay/1 -> Divide1/1
  series cells1/1 -> Product/3

== system untitled/PV Array/PV Module 1/PV Module/Photon current ==
  note: ￼
  T : Inport
  Ir : Inport  Port=2
  Add : Sum  Inputs=+-
  Add1 : Sum
  Constant : Constant  Value=1000
  Divide : Product  Inputs=**/
  Ki : Constant  Value=0.002
  Product : Product
  Scope : Scope
  Tr_value : Constant  Value=25+273.15
  short circuit current : Constant  Value=I_sc
  Iph : Outport
  wires:
  Ki/1 -> Product/1
  Add/1 -> Product/2
  Divide/1 -> Iph/1, Scope/1
  Tr_value/1 -> Add/2
  Product/1 -> Add1/1
  Add1/1 -> Divide/2
  Ir/1 -> Divide/1
  Constant/1 -> Divide/3
  T/1 -> Add/1
  short circuit current/1 -> Add1/2

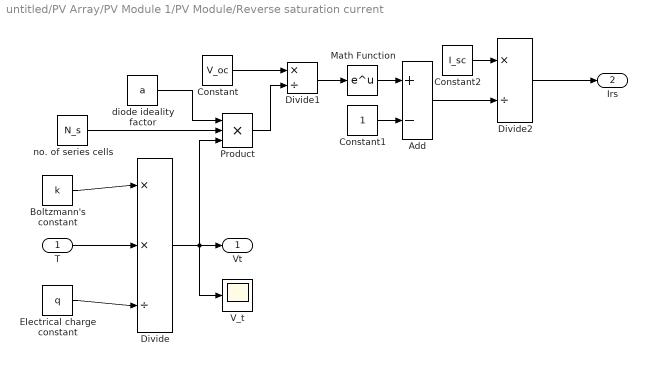
== system untitled/PV Array/PV Module 1/PV Module/Reverse saturation current ==
  T : Inport
  Add : Sum  Inputs=+-
  Boltzmann's constant : Constant  Value=k
  Constant : Constant  Value=V_oc
  Constant1 : Constant
  Constant2 : Constant  Value=I_sc
  Divide : Product  Inputs=**/
  Divide1 : Product  Inputs=*/
  Divide2 : Product  Inputs=*/
  Electrical charge constant : Constant  Value=q
  Math Function : Math  SaturateOnIntegerOverflow=on
  Product : Product  Inputs=3
  V_t : Scope
  diode ideality factor : Constant  Value=a
  no. of series cells : Constant  Value=N_s
  Vt : Outport
  Irs : Outport  Port=2
  wires:
  Product/1 -> Divide1/2
  Divide/1 -> V_t/1, Vt/1, Product/3
  Boltzmann's constant/1 -> Divide/1
  Constant1/1 -> Add/2
  Constant2/1 -> Divide2/1
  Math Function/1 -> Add/1
  Add/1 -> Divide2/2
  diode ideality factor/1 -> Product/1
  Constant/1 -> Divide1/1
  Divide1/1 -> Math Function/1
  T/1 -> Divide/2
  Divide2/1 -> Irs/1
  no. of series cells/1 -> Product/2
  Electrical charge constant/1 -> Divide/3

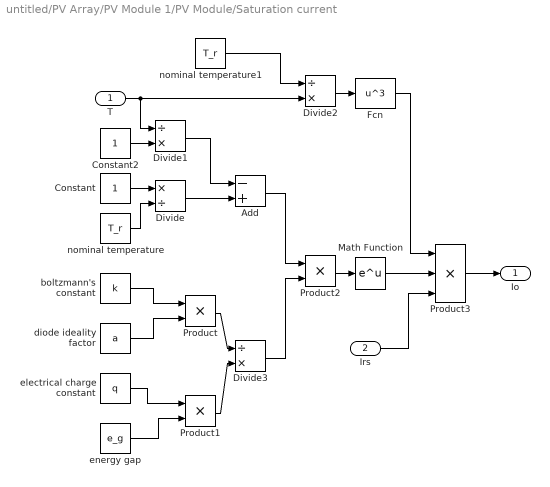
== system untitled/PV Array/PV Module 1/PV Module/Saturation current ==
  T : Inport
  Irs : Inport  Port=2
  Add : Sum  Inputs=-+
  Constant : Constant
  Constant2 : Constant
  Divide : Product  Inputs=*/
  Divide1 : Product  Inputs=/*
  Divide2 : Product  Inputs=/*
  Divide3 : Product  Inputs=/*
  Fcn : Fcn  Expr=u^3
  Math Function : Math  SaturateOnIntegerOverflow=on
  Product : Product
  Product1 : Product
  Product2 : Product
  Product3 : Product  Inputs=3
  boltzmann's constant : Constant  Value=k
  diode ideality factor : Constant  Value=a
  electrical charge constant : Constant  Value=q
  energy gap : Constant  Value=e_g
  nominal temperature : Constant  Value=T_r
  nominal temperature1 : Constant  Value=T_r
  Io : Outport
  wires:
  Divide1/1 -> Add/1
  energy gap/1 -> Product1/2
  Math Function/1 -> Product3/2
  diode ideality factor/1 -> Product/2
  electrical charge constant/1 -> Product1/1
  Product3/1 -> Io/1
  T/1 -> Divide2/2, Divide1/1
  boltzmann's constant/1 -> Product/1
  Constant/1 -> Divide/1
  Add/1 -> Product2/1
  Divide2/1 -> Fcn/1
  Product2/1 -> Math Function/1
  Divide3/1 -> Product2/2
  Fcn/1 -> Product3/1
  Irs/1 -> Product3/3
  Product/1 -> Divide3/1
  nominal temperature1/1 -> Divide2/1
  Product1/1 -> Divide3/2
  Divide/1 -> Add/2
  Constant2/1 -> Divide1/2
  nominal temperature/1 -> Divide/2

== system untitled/PV Array/PV Module 2/PV Module/Current through shunt resistor ==
  V : Inport
  I : Inport  Port=2
  Add : Sum
  Divide : Product  Inputs=*/
  Divide1 : Product  Inputs=*/
  Product : Product
  Product1 : Product
  Unit Delay : UnitDelay  SampleTime=-1  HasFrameUpgradeWarning=on
  no. of parallel cells : Constant  Value=N_p
  no. of series cells : Constant  Value=N_s
  series resistance : Constant  Value=R_s
  shunt resistance : Constant  Value=R_sh
  Ish : Outport
  wires:
  no. of parallel cells/1 -> Product/2
  V/1 -> Product/1
  Divide1/1 -> Ish/1
  Divide/1 -> Add/1
  Product1/1 -> Add/2
  series resistance/1 -> Product1/2
  shunt resistance/1 -> Divide1/2
  no. of series cells/1 -> Divide/2
  Add/1 -> Divide1/1
  Product/1 -> Divide/1
  I/1 -> Unit Delay/1
  Unit Delay/1 -> Product1/1

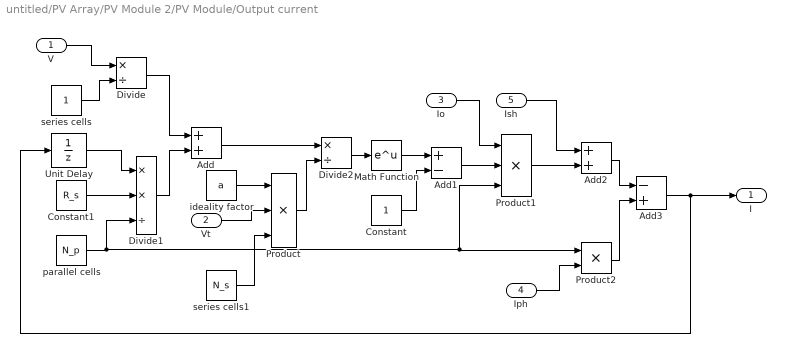
== system untitled/PV Array/PV Module 2/PV Module/Output current ==
  V : Inport
  Vt : Inport  Port=2
  Io : Inport  Port=3
  Iph : Inport  Port=4
  Ish : Inport  Port=5
  Add : Sum
  Add1 : Sum  Inputs=+-
  Add2 : Sum
  Add3 : Sum  Inputs=-+
  Constant : Constant
  Constant1 : Constant  Value=R_s
  Divide : Product  Inputs=*/
  Divide1 : Product  Inputs=**/
  Divide2 : Product  Inputs=*/
  Math Function : Math  SaturateOnIntegerOverflow=on
  Product : Product  Inputs=3
  Product1 : Product  Inputs=3
  Product2 : Product
  Unit Delay : UnitDelay  SampleTime=-1  HasFrameUpgradeWarning=on
  ideality factor : Constant  Value=a
  parallel cells : Constant  Value=N_p
  series cells : Constant
  series cells1 : Constant  Value=N_s
  I : Outport
  wires:
  V/1 -> Divide/1
  Constant/1 -> Add1/2
  parallel cells/1 -> Product2/1, Product1/3, Divide1/3
  Vt/1 -> Product/2
  Add2/1 -> Add3/1
  Ish/1 -> Add2/1
  Product/1 -> Divide2/2
  Divide1/1 -> Add/2
  Divide2/1 -> Math Function/1
  Iph/1 -> Product2/2
  Math Function/1 -> Add1/1
  ideality factor/1 -> Product/1
  Constant1/1 -> Divide1/2
  Add/1 -> Divide2/1
  Product2/1 -> Add3/2
  series cells/1 -> Divide/2
  Divide/1 -> Add/1
  Add1/1 -> Product1/2
  Product1/1 -> Add2/2
  Io/1 -> Product1/1
  Add3/1 -> Unit Delay/1, I/1
  Unit Delay/1 -> Divide1/1
  series cells1/1 -> Product/3

== system untitled/PV Array/PV Module 2/PV Module/Photon current ==
  note: ￼
  T : Inport
  Ir : Inport  Port=2
  Add : Sum  Inputs=+-
  Add1 : Sum
  Constant : Constant  Value=1000
  Divide : Product  Inputs=**/
  Ki : Constant  Value=0.002
  Product : Product
  Scope : Scope
  Tr_value : Constant  Value=25+273.15
  short circuit current : Constant  Value=I_sc
  Iph : Outport
  wires:
  Ki/1 -> Product/1
  Add/1 -> Product/2
  Divide/1 -> Iph/1, Scope/1
  Tr_value/1 -> Add/2
  Product/1 -> Add1/1
  Add1/1 -> Divide/2
  Ir/1 -> Divide/1
  Constant/1 -> Divide/3
  T/1 -> Add/1
  short circuit current/1 -> Add1/2

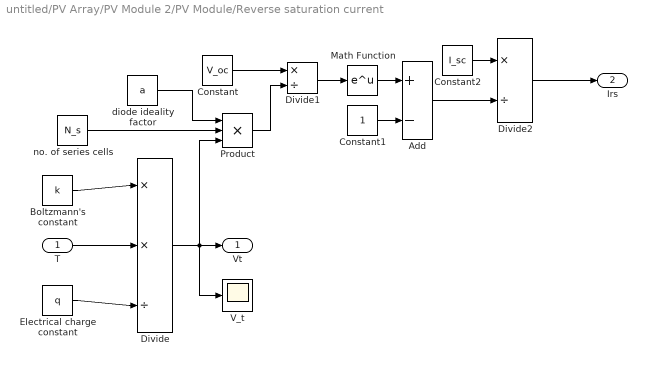
== system untitled/PV Array/PV Module 2/PV Module/Reverse saturation current ==
  T : Inport
  Add : Sum  Inputs=+-
  Boltzmann's constant : Constant  Value=k
  Constant : Constant  Value=V_oc
  Constant1 : Constant
  Constant2 : Constant  Value=I_sc
  Divide : Product  Inputs=**/
  Divide1 : Product  Inputs=*/
  Divide2 : Product  Inputs=*/
  Electrical charge constant : Constant  Value=q
  Math Function : Math  SaturateOnIntegerOverflow=on
  Product : Product  Inputs=3
  V_t : Scope
  diode ideality factor : Constant  Value=a
  no. of series cells : Constant  Value=N_s
  Vt : Outport
  Irs : Outport  Port=2
  wires:
  Product/1 -> Divide1/2
  Divide/1 -> V_t/1, Vt/1, Product/3
  Boltzmann's constant/1 -> Divide/1
  Constant1/1 -> Add/2
  Constant2/1 -> Divide2/1
  Math Function/1 -> Add/1
  Add/1 -> Divide2/2
  diode ideality factor/1 -> Product/1
  Constant/1 -> Divide1/1
  Divide1/1 -> Math Function/1
  T/1 -> Divide/2
  Divide2/1 -> Irs/1
  no. of series cells/1 -> Product/2
  Electrical charge constant/1 -> Divide/3

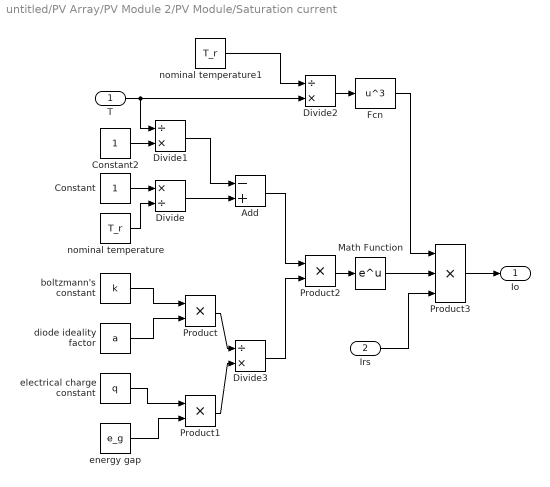
== system untitled/PV Array/PV Module 2/PV Module/Saturation current ==
  T : Inport
  Irs : Inport  Port=2
  Add : Sum  Inputs=-+
  Constant : Constant
  Constant2 : Constant
  Divide : Product  Inputs=*/
  Divide1 : Product  Inputs=/*
  Divide2 : Product  Inputs=/*
  Divide3 : Product  Inputs=/*
  Fcn : Fcn  Expr=u^3
  Math Function : Math  SaturateOnIntegerOverflow=on
  Product : Product
  Product1 : Product
  Product2 : Product
  Product3 : Product  Inputs=3
  boltzmann's constant : Constant  Value=k
  diode ideality factor : Constant  Value=a
  electrical charge constant : Constant  Value=q
  energy gap : Constant  Value=e_g
  nominal temperature : Constant  Value=T_r
  nominal temperature1 : Constant  Value=T_r
  Io : Outport
  wires:
  Divide1/1 -> Add/1
  energy gap/1 -> Product1/2
  Math Function/1 -> Product3/2
  diode ideality factor/1 -> Product/2
  electrical charge constant/1 -> Product1/1
  Product3/1 -> Io/1
  T/1 -> Divide2/2, Divide1/1
  boltzmann's constant/1 -> Product/1
  Constant/1 -> Divide/1
  Add/1 -> Product2/1
  Divide2/1 -> Fcn/1
  Product2/1 -> Math Function/1
  Divide3/1 -> Product2/2
  Fcn/1 -> Product3/1
  Irs/1 -> Product3/3
  Product/1 -> Divide3/1
  nominal temperature1/1 -> Divide2/1
  Product1/1 -> Divide3/2
  Divide/1 -> Add/2
  Constant2/1 -> Divide1/2
  nominal temperature/1 -> Divide/2
